simulink model "hybrid_power"  (R2024b)
settings: Solver=ode45  StartTime=0.0  StopTime=3  MaxStep=0.001  RelTol=1e-3  EnableMultiTasking=on
values from neighbouring files (symbols this model uses):
  Iph_array = Iph*Npar    (= 29.801)    [pvinput.m]
  Isat_array = Isat*Npar    (= 5.8765e-08)    [pvinput.m]
  Rp_array = Rp*Nser/Npar    (= 198.702)    [pvinput.m]
  Rs_array = Rs*Nser/Npar    (= 0.0075996)    [pvinput.m]
  Ts = Ts_Power    (= 1e-06)    [pvinput.m]
  Ts_Control = 100e-6    (= 0.0001)    [pvinput.m]
  Ts_Power = 1e-6    (= 1e-06)    [pvinput.m]
  VT_array = VT*Nser    (= 3.20466023218)    [pvinput.m]
undefined symbols (not defined in the file or in its folder): DiscIntNeverNeededParam, sigbuilder_block
libraries: spsVoltageMeasurementLib x14, spsSeriesRLCBranchLib x8, spsControlledVoltageSourceLib x8, spsGroundLib x5, spsDiodeLib x4, spsIGBTDiodeLib x4, spsParallelRLCBranchLib x3, spsCurrentMeasurementLib x2, simulink x2, spsControlledCurrentSourceLib x2, spsPWMGenerator2LevelLib x1, powerlib_extras x1
settings Model: Creator=Hasin Punno  LastModifiedBy=amank
settings SolverCC: AlgebraicLoopSolver=TrustRegion
settings DataIOCC: LimitDataPoints=on  SaveFormat=Array  SignalLoggingSaveFormat=ModelDataLogs  ReturnWorkspaceOutputs=off
settings OptimizationCC: ExpressionDepthLimit=2147483647  LifeSpan=inf
settings DebuggingCC: UnderspecifiedInitializationDetection=Classic  MergeDetectMultiDrivingBlocksExec=none  SolverPrmCheckMsg=warning  FcnCallInpInsideContextMsg=warning  UnconnectedInputMsg=warning  UnconnectedOutputMsg=warning  UnconnectedLineMsg=warning  StateNameClashWarn=warning  SFUnexpectedBacktrackingDiag=warning  SFNoUnconditionalDefaultTransitionDiag=warning  SFExecutionAtInitializationDiag=none  ArithmeticOperatorsInVariantConditions=warning
settings HardwareCC: ProdBitPerPointer=32  ProdBitPerSizeT=32  ProdBitPerPtrDiffT=32  ProdLargestAtomicFloat=None  ProdIntDivRoundTo=Undefined  ProdEndianess=Unspecified  ProdWordSize=32  ProdHWDeviceType=32-bit Generic
settings ModelReferenceCC: EnableRefExpFcnMdlSchedulingChecks=on  PropagateSignalLabelsOutOfModel=off
settings SFSimCC: SimUseLocalCustomCode=off  CustomCodeUndefinedFunction=UseInterfaceOnly
settings RTWCC: RTWUseLocalCustomCode=off  GPUComputeCapability=3.5
settings CodeAppCC: StateflowObjectComments=on
settings GRTTargetCC: TargetLangStandard=C89/C90 (ANSI)
settings ConfigComp: CovMetricSettings=dw  CovSaveCumulativeToWorkspaceVar=on  CovSaveSingleToWorkspaceVar=on  CovExternalEMLEnable=off  CovSFcnEnable=off
settings SimscapeCC: SimscapeNormalizeSystem=off

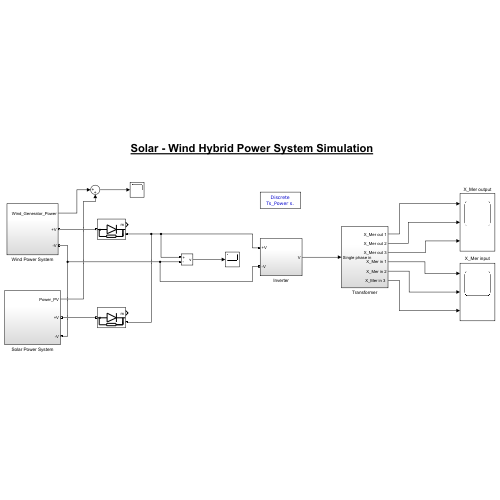
[thumbnail: Simulink's stored preview of the top-level diagram]
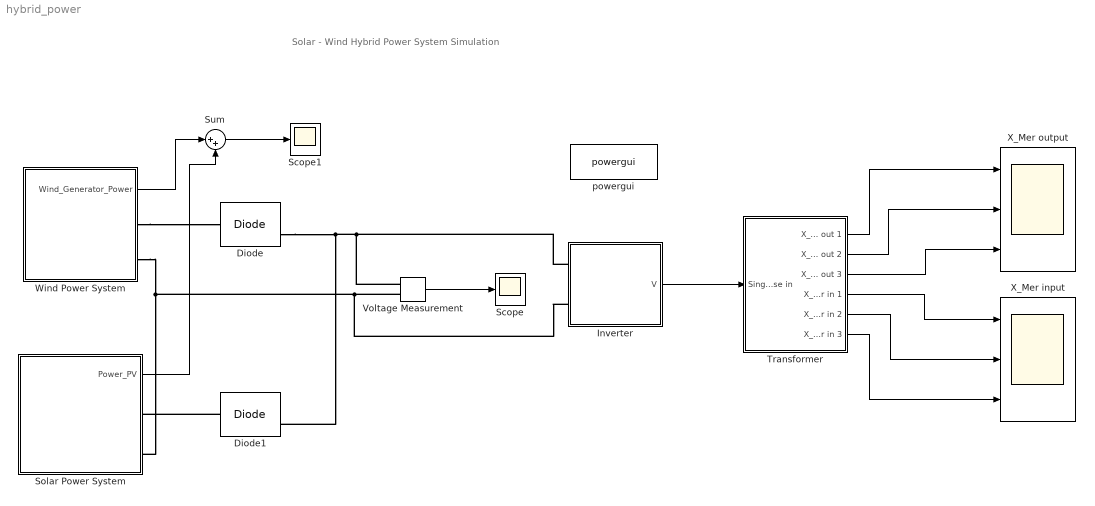
== system hybrid_power ==
  note: Solar - Wind Hybrid Power System Simulation
  Diode : spsDiodeLib/Diode  Ron=0.001  Lon=0  Vf=0.8  IC=0  UseSnubber=off  Rs=500  Cs=1e-9  Measurements=on
  Diode1 : spsDiodeLib/Diode  Ron=0.001  Lon=0  Vf=0.8  IC=0  UseSnubber=off  Rs=500  Cs=1e-9  Measurements=on
  "Inverter " : Subsystem
  Scope : Scope
  Scope1 : Scope
  "Solar Power System " : Subsystem
  Sum : Sum  Inputs=|++
  "Transformer " : Subsystem
  Voltage Measurement : spsVoltageMeasurementLib/Voltage Measurement  PhasorSimulation=off  OutputType=Complex  PSBequivalent=0
  Wind Power System : Subsystem
  X_Mer input : Scope  NumInputPorts=3
  X_Mer output : Scope  NumInputPorts=3
  powergui : spspowerguiLib/powergui  Priority=1  SimulationMode=Discrete  SampleTime=Ts_Power  frequency=60  Iterations=50  frequencyindice=0  Pbase=100e6  ErrMax=1e-4  UnitsV=kV  UnitsW=MW  buscounter=0  FunctionMessages=off  echomessages=off  EnableUseOfTLC=off  CurrentSourceSwitches=off  DisableSnubberDevices=off  DisableRonSwitches=off  DisableVfSwitches=off  DisplayEquations=off  AutomaticDiscreteSolvers=off  SolverType=Tustin  Interpol=off  ExternalGateDelay=off  methode=off  Ts=0  x0status=blocks  SPID=off  SwTol=0  HookPort=off  NonlinearTolerance=1e-4  nMaxIteration=100  ContinueOnMaxIteration=off  RestoreLinks=warning  ResistiveCurrentMeasurement=off  Frange=[0:2:500]  Ylog=off  Xlog=on  ShowGrid=off  save=off  variable=ZData  structure=0  ZoomFFT=on  StartTime=0.0  cycles=1  DisplayStyle=1  fundamental=60  FreqAxis=off  MaxFrequency=1000  frequencyindicesteady=1  RmsSteady=1  display=off
  wires:
  Voltage Measurement/1 -> Scope/1
  Wind Power System/1(Wind_Generator_Power) -> Sum/1
  "Solar Power System "/1(Power_PV) -> Sum/2
  "Inverter "/1(V) -> "Transformer "/1("Single phase in ")
  "Transformer "/1(X_Mer out 1) -> X_Mer output/1
  "Transformer "/2(X_Mer out 2) -> X_Mer output/2
  "Transformer "/3(X_Mer out 3) -> X_Mer output/3
  "Transformer "/4(X_Mer in 1) -> X_Mer input/1
  "Transformer "/5(X_Mer in 2) -> X_Mer input/2
  "Transformer "/6("X_Mer in 3 ") -> X_Mer input/3
  Sum/1 -> Scope1/1
  connections:
  Wind Power System/RConn1 -- Diode/LConn1
  Diode1/LConn1 -- "Solar Power System "/RConn1
  Diode/RConn1 -- Diode1/RConn1 -- Voltage Measurement/LConn1 -- "Inverter "/LConn1
  Wind Power System/RConn2 -- Voltage Measurement/LConn2 -- "Inverter "/LConn2 -- "Solar Power System "/RConn2

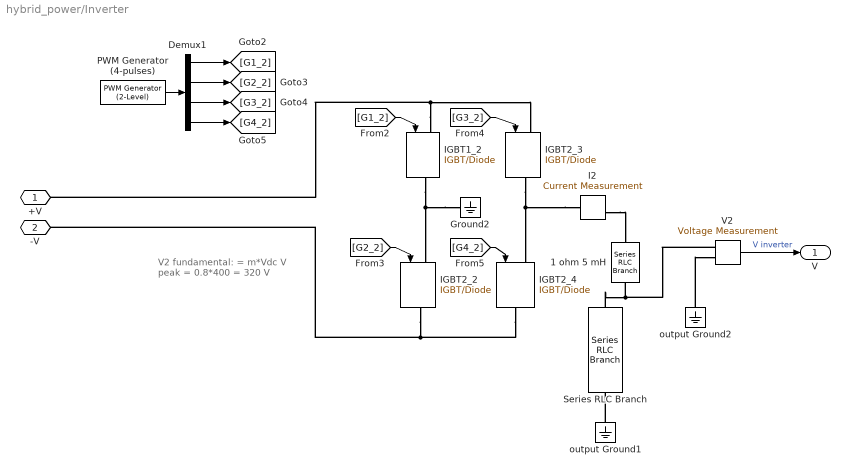
== system hybrid_power/Inverter  ==
  note: V2 fundamental:
      |     = m*Vdc V peak
      |     = 0.8*400
      |     = 320 V
  "1 ohm 5 mH " : spsSeriesRLCBranchLib/Series RLC Branch  LConnTagsString=__new0  RConnTagsString=__new0  BranchType=RL  Resistance=27  Inductance=100e-03  SetiL0=off  InitialCurrent=0  Capacitance=[]  Setx0=off  InitialVoltage=0  Measurements=None
  Demux1 : Demux
  Ground2 : spsGroundLib/Ground  LConnTagsString=a
  I2 : spsCurrentMeasurementLib/Current Measurement  Tag=PoWeRsYsTeMmEaSuReMeNt  PhasorSimulation=off  OutputType=Magnitude  PSBequivalent=0
      settings: AttributesFormatString=\n
  IGBT1_2 : spsIGBTDiodeLib/IGBT//Diode  Ron=1e-3  Rs=1e5  Cs=inf  Measurements=off
  IGBT2_2 : spsIGBTDiodeLib/IGBT//Diode  Ron=1e-3  Rs=1e5  Cs=inf  Measurements=off
  IGBT2_3 : spsIGBTDiodeLib/IGBT//Diode  Ron=1e-3  Rs=1e5  Cs=inf  Measurements=off
  IGBT2_4 : spsIGBTDiodeLib/IGBT//Diode  Ron=1e-3  Rs=1e5  Cs=inf  Measurements=off
  PWM Generator (4-pulses) : spsPWMGenerator2LevelLib/PWM Generator (2-Level)  ModulatorType=Single-phase full-bridge (4 pulses)  ModulatorMode=Unsynchronized  Fc=2000  Pc=0  nF=27  MinMax="[ -1  1 ]"  SamplingTechnique=Natural  ModulatingSignals=on  m=0.8  Freq=50  Phase=0  Ts=5.144e-6  ShowCarrierOutport=off
  Series RLC Branch : spsSeriesRLCBranchLib/Series RLC Branch  LConnTagsString=__new0  RConnTagsString=__new0  BranchType=C  Resistance=1  Inductance=1e-3  SetiL0=off  InitialCurrent=0  Capacitance=100e-6  Setx0=off  InitialVoltage=0  Measurements=None
  V2 : spsVoltageMeasurementLib/Voltage Measurement  Tag=PoWeRsYsTeMmEaSuReMeNt  PhasorSimulation=off  OutputType=Magnitude  PSBequivalent=0
  output Ground1 : spsGroundLib/Ground  LConnTagsString=a
  output Ground2 : spsGroundLib/Ground  LConnTagsString=a
  +V : PMIOPort  Side=Left
  "-V " : PMIOPort  Port=2  Side=Left
  V : Outport
  wires:
  Demux1/4 -> [G4_2]
  V2/1 -> V/1  "V inverter"
  Demux1/2 -> [G2_2]
  [G1_2] -> IGBT1_2/1
  Demux1/3 -> [G3_2]
  PWM Generator (4-pulses)/1 -> Demux1/1
  [G3_2] -> IGBT2_3/1
  Demux1/1 -> [G1_2]
  [G2_2] -> IGBT2_2/1
  [G4_2] -> IGBT2_4/1
  connections:
  I2/LConn1 -- IGBT2_3/RConn1 -- IGBT2_4/LConn1
  V2/LConn1 -- Series RLC Branch/LConn1 -- "1 ohm 5 mH "/RConn1
  Ground2/LConn1 -- IGBT1_2/RConn1 -- IGBT2_2/LConn1
  output Ground2/LConn1 -- V2/LConn2
  I2/RConn1 -- "1 ohm 5 mH "/LConn1
  IGBT1_2/LConn1 -- +V/RConn1 -- IGBT2_3/LConn1
  IGBT2_2/RConn1 -- "-V "/RConn1 -- IGBT2_4/RConn1
  output Ground1/LConn1 -- Series RLC Branch/RConn1

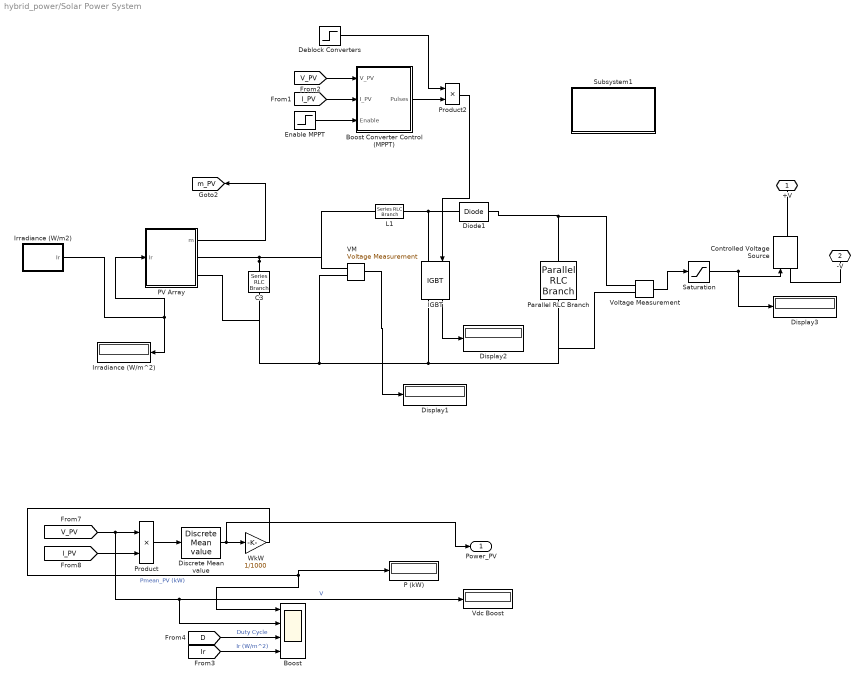
== system hybrid_power/Solar Power System  ==
  Boost : Scope  NumInputPorts=4
  Boost Converter Control (MPPT) : Subsystem
  C3 : spsSeriesRLCBranchLib/Series RLC Branch  LConnTagsString=__new0  RConnTagsString=__new0  BranchType=C  Resistance=1.0  Inductance=1.0  SetiL0=off  InitialCurrent=0  Capacitance=100e-6  Setx0=off  InitialVoltage=0  Measurements=Branch voltage
  Controlled Voltage Source : spsControlledVoltageSourceLib/Controlled Voltage Source  Initialize=on  Source_Type=AC  Amplitude=0  Phase=0  Frequency=0  Measurements=None
  Deblock Converters : Step  Time=0.05  SampleTime=0
  Diode1 : spsDiodeLib/Diode  Ron=1e-4  Lon=0  Vf=0  IC=0  UseSnubber=off  Rs=inf  Cs=inf  Measurements=off
  Discrete Mean value : powerlib_extras/Discrete Measurements/Discrete  Mean value  Freq=60  Vinit=0  Ts=Ts_Control
  Display1 : Display
  Display2 : Display
  Display3 : Display
  Enable MPPT : Step  Time=0.4  SampleTime=0
  IGBT : spsIGBTLib/IGBT  Ron=0.001  Lon=0  Vf=0  Tf=0  Tt=0  IC=0  Rs=1e5  Cs=inf  Measurements=on
  "Irradiance (W/m2) " : Subsystem  Tag=STV Subsys  LoadFcn=sigbuilder_block('load');  StartFcn=sigbuilder_block('start');  StopFcn=sigbuilder_block('stop');  ClipboardFcn=sigbuilder_block('clipboard');  mask(Sigbuilder block){tuvar=[0:10]}
      mask help: Sigbuilder GUI
      mask init:
      | if ~strcmp(get_param(bdroot(gcbh),'SimulationStatus'),'stopped') tuvar = sigbuilder_block('maskInit'); end
      settings: CopyFcn=sigbuilder_block('copy');  DeleteFcn=sigbuilder_block('delete');  ModelCloseFcn=sigbuilder_block('modelClose');  PreSaveFcn=sigbuilder_block('preSave');  PauseFcn=sigbuilder_block('pause')  ContinueFcn=sigbuilder_block('continue')  NameChangeFcn=sigbuilder_block('namechange');  OpenFcn=sigbuilder_block('open',[9 39 954 473.25 ]);  CloseFcn=sigbuilder_block('close');
      mask Display: plot(0, 0, 100, 100,[2, 2, 32, 32, 2], [68, 8, 8, 68, 68],[32, 2], [38, 38], [32, 19, 2],[53, 60, 44], [32, 17, 17, 2],[16, 16, 31, 31]);txt = getActiveGroup(gcbh);text(2, 100, txt,'verticalAlignment', 'top');
  Irradiance (W/m^2) : Display
      settings: Format=bank  Decimation=1000
  L1 : spsSeriesRLCBranchLib/Series RLC Branch  LConnTagsString=__new0  RConnTagsString=__new0  BranchType=RL  Resistance=0.005  Inductance=5e-3  SetiL0=off  InitialCurrent=0  Capacitance=1e-6  Setx0=off  InitialVoltage=0  Measurements=None
  "P (kW) " : Display
      settings: Format=bank  Decimation=2000
  PV Array : Subsystem
  Parallel RLC Branch : spsParallelRLCBranchLib/Parallel RLC Branch  LConnTagsString=a  RConnTagsString=__new0  BranchType=RC  Resistance=1e3  Inductance=1e-3  SetiL0=off  InitialCurrent=0  Capacitance=1e-6  Setx0=off  InitialVoltage=0  Measurements=None
  Product : Product  RndMeth=Zero
  Product2 : Product  RndMeth=Zero
  Saturation : Saturate  UpperLimit=48  LowerLimit=0
  Subsystem1 : Subsystem
      mask Display: disp('Measurements')
  VM : spsVoltageMeasurementLib/Voltage Measurement  PhasorSimulation=off  OutputType=Complex  PSBequivalent=0
  Vdc Boost : Display
      settings: Format=bank  Decimation=2000
  Voltage Measurement : spsVoltageMeasurementLib/Voltage Measurement  PhasorSimulation=off  OutputType=Complex  PSBequivalent=0
  WkW : Gain  Gain=1/1000
  +V : PMIOPort  Side=Right
  -V : PMIOPort  Port=2  Side=Right
  Power_PV : Outport
  tag scope: m_PV=global
  wires:
  Voltage Measurement/1 -> Saturation/1
  Saturation/1 -> Controlled Voltage Source/1, Display3/1
  IGBT/1 -> Display2/1
  PV Array/1(m) -> [m_PV]
  [D] -> Boost/3  "Duty Cycle"
  [V_PV] -> Vdc Boost/1, Boost/2, Product/1  "V"
  VM/1 -> Display1/1
  "Irradiance (W/m2) "/1(Ir) -> Irradiance (W/m^2)/1, PV Array/1(Ir)
  [Ir] -> Boost/4  "Ir (W/m^2)"
  Deblock Converters/1 -> Product2/1
  Product2/1 -> IGBT/1
  Enable MPPT/1 -> Boost Converter Control (MPPT)/3(Enable)
  Boost Converter Control (MPPT)/1(Pulses) -> Product2/2
  [I_PV] -> Boost Converter Control (MPPT)/2(I_PV)
  [V_PV] -> Boost Converter Control (MPPT)/1(V_PV)
  Discrete Mean value/1 -> Power_PV/1, WkW/1
  WkW/1 -> "P (kW) "/1, Boost/1  "Pmean_PV (kW)"
  [I_PV] -> Product/2
  Product/1 -> Discrete Mean value/1
  connections:
  Controlled Voltage Source/LConn1 -- -V/RConn1
  +V/RConn1 -- Controlled Voltage Source/RConn1
  IGBT/LConn1 -- L1/RConn1 -- Diode1/LConn1
  C3/LConn1 -- PV Array/RConn1 -- L1/LConn1 -- VM/LConn1
  VM/LConn2 -- PV Array/RConn2 -- C3/RConn1 -- IGBT/RConn1 -- Parallel RLC Branch/RConn1 -- Voltage Measurement/LConn2
  Voltage Measurement/LConn1 -- Parallel RLC Branch/LConn1 -- Diode1/RConn1

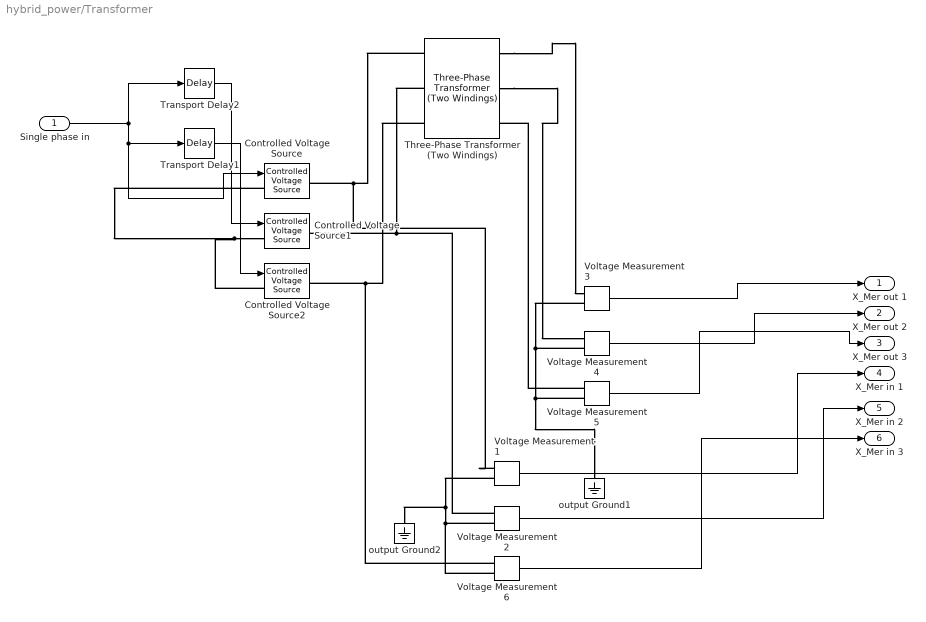
== system hybrid_power/Transformer  ==
  "Single phase in " : Inport
  Controlled Voltage Source : spsControlledVoltageSourceLib/Controlled Voltage Source  Initialize=on  Source_Type=AC  Amplitude=48  Phase=0  Frequency=50  Measurements=Voltage
  Controlled Voltage Source1 : spsControlledVoltageSourceLib/Controlled Voltage Source  Initialize=on  Source_Type=AC  Amplitude=48  Phase=120  Frequency=50  Measurements=Voltage
  Controlled Voltage Source2 : spsControlledVoltageSourceLib/Controlled Voltage Source  Initialize=on  Source_Type=AC  Amplitude=48  Phase=240  Frequency=50  Measurements=None
  Three-Phase Transformer (Two Windings) : spsThreePhaseTransformerTwoWindingsLib/Three-Phase Transformer (Two Windings)  Winding1Connection=Yg  Winding2Connection=Yg  CoreType=Three single-phase transformers  SetSaturation=off  Hysteresis=off  DataFile='hysteresis'  SetInitialFlux=off  Measurements=None  UNITS=SI  NominalPower=[9444 , 50 ]  Winding1=[48 0.018432 0.00023468]  Winding2=[460 1.62 0.020626]  Rm=4608  Lm=14.668  L0=0.5  Saturation=[0 0;0.010206 1.2475e+05;4.2526 1.5802e+05]  InitialFluxes=[83168 -83168 72773]  BreakLoop=off  DiscreteSolver=Trapezoidal iterative  DataType=on  TransfoNumber=1
  Transport Delay1 : TransportDelay  DelayTime=0.013333  BufferSize=10240
  Transport Delay2 : TransportDelay  DelayTime=6.6667e-3  BufferSize=10240
  Voltage Measurement{1..6} (6 alike) : spsVoltageMeasurementLib/Voltage Measurement  PhasorSimulation=off  OutputType=Complex  PSBequivalent=0
  output Ground1 : spsGroundLib/Ground  LConnTagsString=a
  output Ground2 : spsGroundLib/Ground  LConnTagsString=a
  X_Mer out 1 : Outport
  X_Mer out 2 : Outport  Port=2
  X_Mer out 3 : Outport  Port=3
  X_Mer in 1 : Outport  Port=4
  X_Mer in 2 : Outport  Port=5
  "X_Mer in 3 " : Outport  Port=6
  wires:
  Voltage Measurement5/1 -> X_Mer out 3/1
  Voltage Measurement4/1 -> X_Mer out 2/1
  Transport Delay1/1 -> Controlled Voltage Source2/1
  "Single phase in "/1 -> Controlled Voltage Source/1, Transport Delay1/1, Transport Delay2/1
  Transport Delay2/1 -> Controlled Voltage Source1/1
  Voltage Measurement1/1 -> X_Mer in 1/1
  Voltage Measurement6/1 -> "X_Mer in 3 "/1
  Voltage Measurement2/1 -> X_Mer in 2/1
  Voltage Measurement3/1 -> X_Mer out 1/1
  connections:
  Three-Phase Transformer (Two Windings)/RConn1 -- Voltage Measurement3/LConn1
  Controlled Voltage Source/LConn1 -- Controlled Voltage Source2/LConn1 -- Controlled Voltage Source1/LConn1
  Three-Phase Transformer (Two Windings)/LConn1 -- Voltage Measurement1/LConn1 -- Controlled Voltage Source/RConn1
  Voltage Measurement5/LConn1 -- Three-Phase Transformer (Two Windings)/RConn3
  Three-Phase Transformer (Two Windings)/RConn2 -- Voltage Measurement4/LConn1
  Three-Phase Transformer (Two Windings)/LConn2 -- Controlled Voltage Source1/RConn1 -- Voltage Measurement2/LConn1
  Voltage Measurement6/LConn2 -- Voltage Measurement1/LConn2 -- output Ground2/LConn1 -- Voltage Measurement2/LConn2
  Three-Phase Transformer (Two Windings)/LConn3 -- Voltage Measurement6/LConn1 -- Controlled Voltage Source2/RConn1
  Voltage Measurement5/LConn2 -- Voltage Measurement3/LConn2 -- Voltage Measurement4/LConn2 -- output Ground1/LConn1

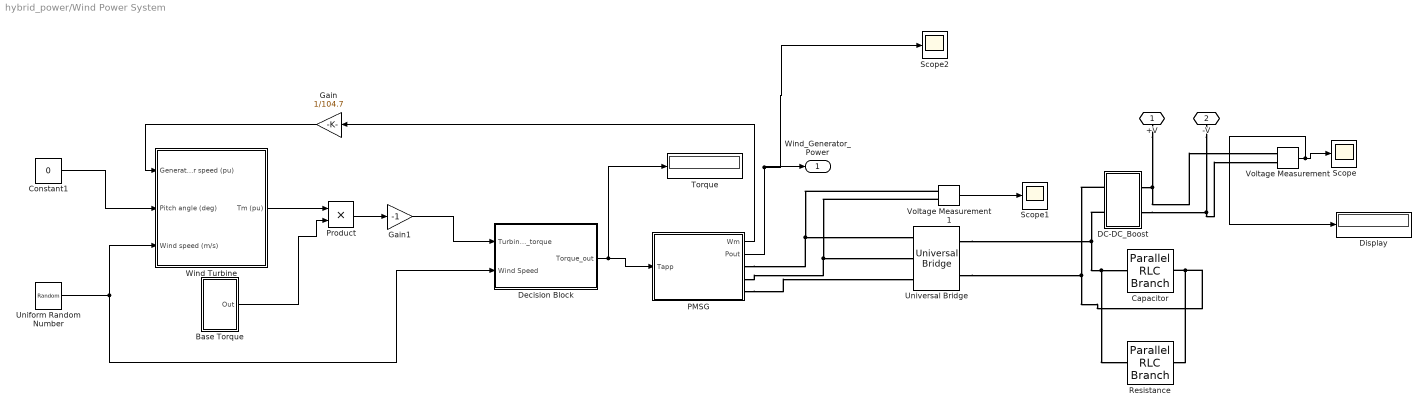
== system hybrid_power/Wind Power System ==
  Base Torque : Subsystem  mask{P=8500, w=104.7}
      mask prompts: P "Base Power"; w "Base speed (rad/s)"
  Capacitor : spsParallelRLCBranchLib/Parallel RLC Branch  LConnTagsString=a  RConnTagsString=__new0  BranchType=C  Resistance=1  Inductance=1e-3  SetiL0=off  InitialCurrent=0  Capacitance=4.8e-4  Setx0=off  InitialVoltage=0  Measurements=None
  Constant1 : Constant  Value=0
  DC-DC_Boost : Subsystem
  Decision Block : Subsystem
  Display : Display
  Gain : Gain  Gain=1/104.7
  Gain1 : Gain  Gain=-1
  PMSG : Subsystem  mask{f=50, p=6, Xs=1, Nc=30, loss=1000, phi=0.0207862}
      mask prompts: f "Frequency(Hz)"; p "Pole"; Xs "Synchronous Reactance(Ohm)"; Nc "Number of turns"; loss "Mechanical Loss(Watt)"; phi "field(Wb-m^2)"
  Product : Product
  Resistance : spsParallelRLCBranchLib/Parallel RLC Branch  LConnTagsString=a  RConnTagsString=__new0  BranchType=R  Resistance=1000  Inductance=1e-3  SetiL0=off  InitialCurrent=0  Capacitance=1  Setx0=off  InitialVoltage=0  Measurements=None
  Scope : Scope
  Scope1 : Scope
  Scope2 : Scope
  Torque : Display
  Uniform Random Number : UniformRandomNumber  Minimum=12  Maximum=13  SampleTime=0.01
  Universal Bridge : spsUniversalBridgeLib/Universal Bridge  Arms=3  SnubberResistance=1e5  SnubberCapacitance=inf  Device=Diodes  Ron=1e-3  Lon=0  ForwardVoltages="[  0  0  ]"  ForwardVoltage=0  GTOparameters=[ 10e-6 , 20e-6 ]  IGBTparameters=[ 1e-6 , 2e-6 ]  Measurements=None  Measurements_2=None  converterType=Rectifier
  Voltage Measurement : spsVoltageMeasurementLib/Voltage Measurement  PhasorSimulation=off  OutputType=Complex  PSBequivalent=0
  Voltage Measurement1 : spsVoltageMeasurementLib/Voltage Measurement  PhasorSimulation=off  OutputType=Complex  PSBequivalent=0
  Wind Turbine : Subsystem  AncestorBlock=re_lib/Wind Generation/Wind Turbine  DialogController=POWERSYS.PowerSysDialog  mask(Wind Turbine){Pnom=8500, Pelec_base=8500/0.9, wind_base=12, P_wind_base=0.8, speed_nom=1, pitch_angle=0, c1_c6=[0.51763          116          0.4            5           21     0.006795], cp_nom=0.48, lambda_nom=8.1}
      mask prompts: Pnom "Nominal mechanical output power (W):"; Pelec_base "Base power of the electrical generator (VA):"; wind_base "Base wind speed (m/s):"; P_wind_base "Maximum power at base wind speed (pu of nominal mechanical power):"; speed_nom "Base rotational speed (p.u. of base generator speed):"; pitch_angle "Pitch angle beta to display wind-turbine power characteristics (beta >=0)  (deg):"
      mask help:
      | This block implements a variable pitch wind turbine model. The performance coefficient Cp of the turbine is the mechanical output power of the turbine divided by wind power and a function of wind speed, rotational speed, and pitch angle (beta). Cp reaches its maximum value at zero beta. Select the wind-turbine power characteristics display to plot the turbine characteristics at the specified pitch angle.
      |
      | The first input is the generator speed in per unit of the generator base speed. For a synchronous or asynchronous generator, the base speed is the synchronous speed. For a permanent-magnet generator, the base speed is defined as the speed producing nominal voltage at  no load. The second input is the blade pitch angle (beta) in degrees. The third input is the wind speed in m/s.
      |
      | The output is the torque applied to the generator shaft in per unit of the generator ratings.
      |
      | The turbine inertia must be added to the generator inertia.
      mask init:
      | c1=c1_c6(1);c2=c1_c6(2);c3=c1_c6(3);c4=c1_c6(4);c5=c1_c6(5);c6=c1_c6(6);
      | if ~(wind_base>0)
      |     error(message('physmod:powersys:common:GreaterThan',getfullname(gcbh),'Base wind speed (m/s)',0));
      | end
      | 
      | power_initmask();
      mask Help: helpview(psbhelp);
      mask DialogControl DisplayTurbChar Prompt: Display wind turbine power characteristics
      mask DialogControl DisplayTurbChar Callback: WindTurbinePlot(gcb)
      mask Display: disp('');
  +V : PMIOPort  Side=Right
  -V : PMIOPort  Port=2  Side=Right
  Wind_Generator_Power : Outport
  wires:
  Gain/1 -> Wind Turbine/1(Generator speed (pu))
  Voltage Measurement/1 -> Display/1, Scope/1
  Base Torque/1(Out) -> Product/2
  Product/1 -> Gain1/1
  PMSG/1(Wm) -> Gain/1
  Wind Turbine/1(Tm (pu)) -> Product/1
  Decision Block/1(Torque_out) -> Torque/1, PMSG/1(Tapp)
  Gain1/1 -> Decision Block/1(Turbine_torque)
  Voltage Measurement1/1 -> Scope1/1
  Constant1/1 -> Wind Turbine/2(Pitch angle (deg))
  PMSG/2(Pout) -> Scope2/1, Wind_Generator_Power/1
  Uniform Random Number/1 -> Decision Block/2(Wind Speed), Wind Turbine/3(Wind speed (m/s))
  connections:
  DC-DC_Boost/RConn1 -- Voltage Measurement/LConn1 -- +V/RConn1
  DC-DC_Boost/RConn2 -- Voltage Measurement/LConn2 -- -V/RConn1
  Universal Bridge/RConn1 -- Capacitor/LConn1 -- Resistance/LConn1 -- DC-DC_Boost/LConn2
  Universal Bridge/RConn2 -- Resistance/RConn1 -- Capacitor/RConn1 -- DC-DC_Boost/LConn1
  PMSG/RConn1 -- Voltage Measurement1/LConn1 -- Universal Bridge/LConn1
  PMSG/RConn2 -- Voltage Measurement1/LConn2 -- Universal Bridge/LConn2
  PMSG/RConn3 -- Universal Bridge/LConn3

== system hybrid_power/Solar Power System /Boost Converter Control (MPPT) ==
  V_PV : Inport
  I_PV : Inport  Port=2
  Enable : Inport  Port=3
  Add : Sum  Inputs=+-
  Initial Duty Cycle : Constant  Value=0.5
  MPPT : Subsystem
  Pulse Generator : Subsystem  mask{Freq=5000}
      mask prompts: Freq "Frequency (Hz)"
  Saturation : Saturate  UpperLimit=1  LowerLimit=0
  Pulses : Outport
  tag scope: D=global
  wires:
  Initial Duty Cycle/1 -> Add/1
  MPPT/1(Delta_D) -> Add/2
  Add/1 -> Saturation/1  "D"
  Saturation/1 -> Pulse Generator/1(D), [D]
  Enable/1 -> MPPT/3(on/off)
  Pulse Generator/1(Pulses) -> Pulses/1
  I_PV/1 -> MPPT/2(I_PV)
  V_PV/1 -> MPPT/1(V_PV)

== system hybrid_power/Solar Power System /Irradiance (W//m2)  ==
  Demux : Demux  Tag=STV Demux  Outputs=1
      settings: DisplayOption=none
  FromWs : FromWorkspace  Tag=STV FromWs  VariableName=tuvar
      SigBuilderData=|
      | common.afterFinalStr = 'Extrapolate'
      | common.sampleTime = '0'
      | dataSet(1).timeRange = [0 1]
      | dataSet(1).name = 'Constant Irradiance'
      | dataSet(2).timeRange = [0 1]
      | dataSet(2).name = 'Step Irradiance'
      | dataSet(3).timeRange = [0 3]
      | dataSet(3).name = 'Ramp-up/down Irradiance'
      | sbobj.Groups(1).Name = 'Constant Irradiance'
      | sbobj.Groups(1).Signals.Name = 'Ir'
      | sbobj.Groups(1).Signals.XData = [0 1]
      | sbobj.Groups(1).Signals.YData = [1000 1000]
      | sbobj.Groups(1).TimeRange = [0 1]
      | sbobj.Groups(2).Name = 'Step Irradiance'
      | sbobj.Groups(2).Signals.Name = 'Ir'
      | sbobj.Groups(2).Signals.XData = [0 0.501 0.51 0.69 0.7 1]
      | sbobj.Groups(2).Signals.YData = [1000 1000 250 250 1000 1000]
      | sbobj.Groups(2).TimeRange = [0 1]
      | sbobj.Groups(3).Name = 'Ramp-up/down Irradiance'
      | sbobj.Groups(3).Signals.Name = 'Ir'
      | sbobj.Groups(3).Signals.XData = [0 0.7 1.2 1.2 1.5 2 2.3 2.35 2.65 2.7 3]
      | sbobj.Groups(3).Signals.YData = [1000 1000 590 595 595 1000 1000 250 250 1000 1000]
      | sbobj.Groups(3).TimeRange = [0 3]
  Ir : Outport  Tag=STV Outport
  wires:
  Demux/1 -> Ir/1
  FromWs/1 -> Demux/1

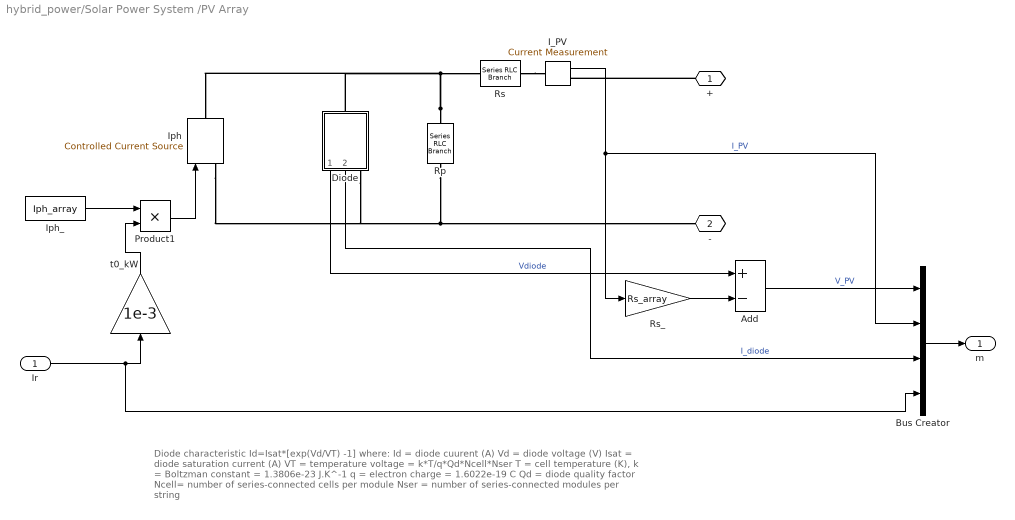
== system hybrid_power/Solar Power System /PV Array ==
  note: Diode characteristic
      | Id=Isat*[exp(Vd/VT) -1]
      |
      | where:
      | Id = diode cuurent (A)
      | Vd = diode voltage (V)
      | Isat = diode saturation current (A)
      | VT = temperature voltage = k*T/q*Qd*Ncell*Nser
      |
      | T = cell temperature (K),
      | k = Boltzman constant = 1.3806e-23 J.K^-1
      | q = electron charge = 1.6022e-19 C
      | Qd = diode quality factor
      | Ncell= number of series-connected cells per module
      | Nser = number of series-connected modules per string
  Ir : Inport
  Add : Sum  Inputs=+-
  Bus Creator : BusCreator  Inputs=4
  Diode : Subsystem
      mask Display:
      | plot(-75,-50,100,150, [-15 -15 43 -15 -15 -75],[50 8 50 92 50 50], ...
      |     [43 43],[8 94],[100 43], [50 50])
  I_PV : spsCurrentMeasurementLib/Current Measurement  PhasorSimulation=off  OutputType=Complex  PSBequivalent=0
  Iph : spsControlledCurrentSourceLib/Controlled Current Source  Initialize=on  Source_Type=AC  Amplitude=0  Phase=0  Frequency=0  Measurements=None
  Iph_ : Constant  Value=Iph_array
  Product1 : Product  Inputs=**  RndMeth=Zero
  Rp : spsSeriesRLCBranchLib/Series RLC Branch  LConnTagsString=__new0  RConnTagsString=__new0  BranchType=R  Resistance=Rp_array  Inductance=1e-3  SetiL0=off  InitialCurrent=0  Capacitance=1e-6  Setx0=off  InitialVoltage=0  Measurements=Branch current
  Rs : spsSeriesRLCBranchLib/Series RLC Branch  LConnTagsString=__new0  RConnTagsString=__new0  BranchType=R  Resistance=Rs_array  Inductance=1e-3  SetiL0=off  InitialCurrent=0  Capacitance=1e-6  Setx0=off  InitialVoltage=0  Measurements=None
  Rs_ : Gain  Gain=Rs_array
  t0_kW : Gain  Gain=1e-3
  + : PMIOPort  Side=Right
  - : PMIOPort  Port=2  Side=Right
  m : Outport
  wires:
  I_PV/1 -> Bus Creator/2, Rs_/1  "I_PV"
  Bus Creator/1 -> m/1
  Rs_/1 -> Add/2
  Diode/1(Vdiode) -> Add/1  "Vdiode"
  Diode/2(Idiode) -> Bus Creator/3  "I_diode"
  Add/1 -> Bus Creator/1  "V_PV"
  t0_kW/1 -> Product1/2
  Product1/1 -> Iph/1
  Iph_/1 -> Product1/1
  Ir/1 -> Bus Creator/4, t0_kW/1
  connections:
  +/RConn1 -- I_PV/RConn1
  Rs/LConn1 -- I_PV/LConn1
  Rp/LConn1 -- Rs/RConn1 -- Iph/RConn1 -- Diode/LConn1
  Rp/RConn1 -- Diode/RConn1 -- Iph/LConn1 -- -/RConn1

== system hybrid_power/Solar Power System /Subsystem1 ==
  Bus Selector : BusSelector  OutputSignals=V_PV,I_PV,I_diode,signal4
  PV : Scope  NumInputPorts=3
  tag scope: I_PV=global, Idiode_PV=global, Ir=global, V_PV=global
  wires:
  [V_PV] -> PV/1  "V_PV"
  [I_PV] -> PV/2  "I_PV"
  [Idiode_PV] -> PV/3  "Idiode_PV"
  [m_PV] -> Bus Selector/1
  Bus Selector/1 -> [V_PV]  "<V_PV>"
  Bus Selector/2 -> [I_PV]  "<I_PV>"
  Bus Selector/3 -> [Idiode_PV]  "<I_diode>"
  Bus Selector/4 -> [Ir]  "<signal4>"

== system hybrid_power/Wind Power System/Base Torque ==
  Base Power : Constant  Value=P
  Base speed(rad/s) : Constant  Value=w
  Divide : Product  Inputs=*/
  Out : Outport
  wires:
  Divide/1 -> Out/1
  Base speed(rad/s)/1 -> Divide/2
  Base Power/1 -> Divide/1

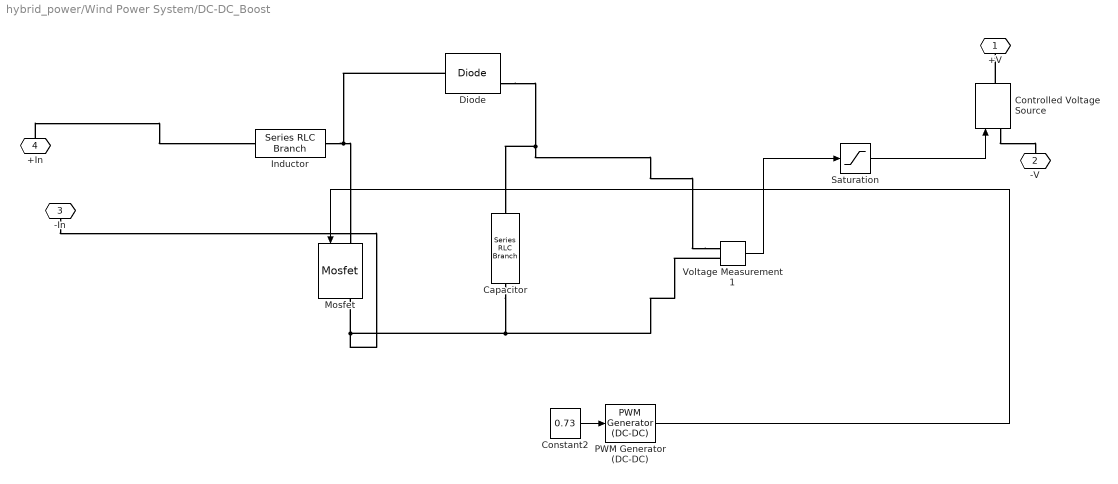
== system hybrid_power/Wind Power System/DC-DC_Boost ==
  Capacitor : spsSeriesRLCBranchLib/Series RLC Branch  LConnTagsString=__new0  RConnTagsString=__new0  BranchType=C  Resistance=1  Inductance=1e-3  SetiL0=off  InitialCurrent=0  Capacitance=33e-6  Setx0=off  InitialVoltage=0  Measurements=None
  Constant2 : Constant  Value=0.73
  Controlled Voltage Source : spsControlledVoltageSourceLib/Controlled Voltage Source  Initialize=on  Source_Type=AC  Amplitude=0  Phase=0  Frequency=0  Measurements=None
  Diode : spsDiodeLib/Diode  Ron=0.001  Lon=0  Vf=0.8  IC=0  UseSnubber=off  Rs=500  Cs=250e-9  Measurements=on
  Inductor : spsSeriesRLCBranchLib/Series RLC Branch  LConnTagsString=__new0  RConnTagsString=__new0  BranchType=L  Resistance=1  Inductance=1e-3  SetiL0=off  InitialCurrent=0  Capacitance=1e-6  Setx0=off  InitialVoltage=0  Measurements=None
  Mosfet : spsMosfetLib/Mosfet  Ron=0.001  Lon=0  Rd=0.001  Vfd=0  IC=0  Rs=1e5  Cs=inf  Measurements=on
  PWM Generator (DC-DC) : spsPWMGeneratorDCDCLib/PWM Generator (DC-DC)  Fsw=25000  Ts=0
  Saturation : Saturate  UpperLimit=48  LowerLimit=0
  Voltage Measurement1 : spsVoltageMeasurementLib/Voltage Measurement  PhasorSimulation=off  OutputType=Complex  PSBequivalent=0
  +V : PMIOPort  Side=Right
  -V : PMIOPort  Port=2  Side=Right
  -In : PMIOPort  Port=3  Side=Left
  +In : PMIOPort  Port=4  Side=Left
  wires:
  Saturation/1 -> Controlled Voltage Source/1
  Constant2/1 -> PWM Generator (DC-DC)/1
  Voltage Measurement1/1 -> Saturation/1
  PWM Generator (DC-DC)/1 -> Mosfet/1
  connections:
  Inductor/RConn1 -- Mosfet/LConn1 -- Diode/LConn1
  +In/RConn1 -- Inductor/LConn1
  Mosfet/RConn1 -- Voltage Measurement1/LConn2 -- Capacitor/RConn1 -- -In/RConn1
  Voltage Measurement1/LConn1 -- Capacitor/LConn1 -- Diode/RConn1
  Controlled Voltage Source/LConn1 -- -V/RConn1
  Controlled Voltage Source/RConn1 -- +V/RConn1

== system hybrid_power/Wind Power System/Decision Block ==
  Turbine_torque : Inport
  Wind Speed : Inport  Port=2
  Switch : Switch  Criteria=u2 > Threshold  SaturateOnIntegerOverflow=off  InputSameDT=off
  Switch1 : Switch  Criteria=u2 > Threshold  Threshold=30  SaturateOnIntegerOverflow=off  InputSameDT=off
  zero : Constant  Value=0
  Torque_out : Outport
  wires:
  Switch1/1 -> Torque_out/1
  Switch/1 -> Switch1/3
  Turbine_torque/1 -> Switch/1, Switch/2
  zero/1 -> Switch1/1, Switch/3
  Wind Speed/1 -> Switch1/2

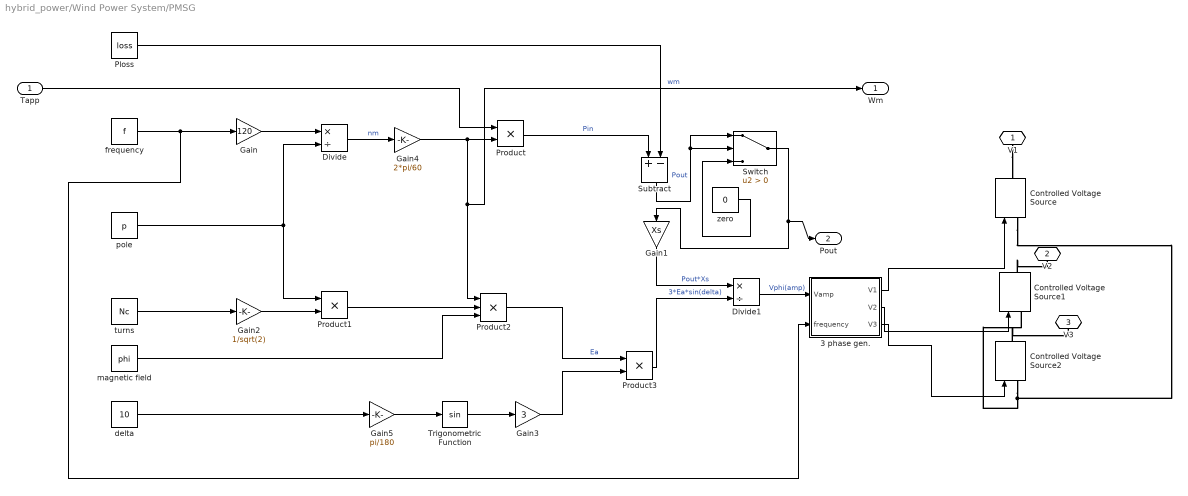
== system hybrid_power/Wind Power System/PMSG ==
  Tapp : Inport
  3 phase gen. : Subsystem
  Controlled Voltage Source : spsControlledVoltageSourceLib/Controlled Voltage Source  Initialize=on  Source_Type=AC  Amplitude=0  Phase=0  Frequency=0  Measurements=None
  Controlled Voltage Source1 : spsControlledVoltageSourceLib/Controlled Voltage Source  Initialize=on  Source_Type=AC  Amplitude=0  Phase=0  Frequency=0  Measurements=None
  Controlled Voltage Source2 : spsControlledVoltageSourceLib/Controlled Voltage Source  Initialize=on  Source_Type=AC  Amplitude=0  Phase=0  Frequency=0  Measurements=None
  Divide : Product  Inputs=*/
  Divide1 : Product  Inputs=*/
  Gain : Gain  Gain=120
  Gain1 : Gain  Gain=Xs
  Gain2 : Gain  Gain=1/sqrt(2)
  Gain3 : Gain  Gain=3
  Gain4 : Gain  Gain=2*pi/60
  Gain5 : Gain  Gain=pi/180
  Ploss : Constant  Value=loss
  Product : Product  RndMeth=Zero
  Product1 : Product  RndMeth=Zero
  Product2 : Product  Inputs=3  RndMeth=Zero
  Product3 : Product  RndMeth=Zero
  Subtract : Sum  Inputs=+-
  Switch : Switch  Criteria=u2 > Threshold  SaturateOnIntegerOverflow=off  InputSameDT=off
  Trigonometric Function : Trigonometry
  delta : Constant  Value=10
  frequency : Constant  Value=f
  magnetic field : Constant  Value=phi
  pole : Constant  Value=p
  turns : Constant  Value=Nc
  zero : Constant  Value=0
  V1 : PMIOPort  Side=Right
  V2 : PMIOPort  Port=2  Side=Right
  V3 : PMIOPort  Port=3  Side=Right
  Wm : Outport
  Pout : Outport  Port=2
  wires:
  Gain/1 -> Divide/1
  turns/1 -> Gain2/1
  Gain2/1 -> Product1/2
  Product1/1 -> Product2/2
  Trigonometric Function/1 -> Gain3/1
  Gain3/1 -> Product3/2
  Gain1/1 -> Divide1/1  "Pout*Xs"
  Product3/1 -> Divide1/2  "3*Ea*sin(delta)"
  delta/1 -> Gain5/1
  Gain5/1 -> Trigonometric Function/1
  Divide/1 -> Gain4/1  "nm"
  frequency/1 -> Gain/1, 3 phase gen./2(frequency)
  Gain4/1 -> Product/2, Product2/1, Wm/1  "wm"
  Tapp/1 -> Product/1
  pole/1 -> Divide/2, Product1/1
  Product/1 -> Subtract/1  "Pin"
  Ploss/1 -> Subtract/2
  Subtract/1 -> Switch/1, Switch/2  "Pout"
  magnetic field/1 -> Product2/3
  Product2/1 -> Product3/1  "Ea"
  Divide1/1 -> 3 phase gen./1(Vamp)  "Vphi(amp)"
  3 phase gen./1(V1) -> Controlled Voltage Source/1
  3 phase gen./2(V2) -> Controlled Voltage Source1/1
  3 phase gen./3(V3) -> Controlled Voltage Source2/1
  zero/1 -> Switch/3
  Switch/1 -> Pout/1, Gain1/1
  connections:
  Controlled Voltage Source2/LConn1 -- Controlled Voltage Source/LConn1 -- Controlled Voltage Source1/LConn1
  V1/RConn1 -- Controlled Voltage Source/RConn1
  Controlled Voltage Source1/RConn1 -- V2/RConn1
  Controlled Voltage Source2/RConn1 -- V3/RConn1

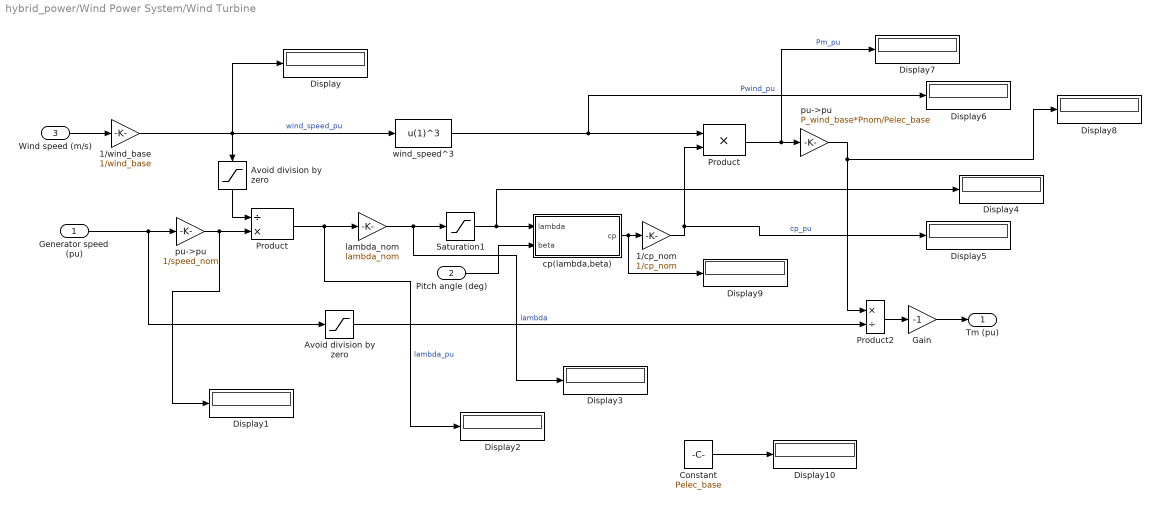
== system hybrid_power/Wind Power System/Wind Turbine ==
  Generator speed (pu) : Inport
  Pitch angle (deg) : Inport  Port=2
  Wind speed (m/s) : Inport  Port=3
  1/cp_nom : Gain  Gain=1/cp_nom  SaturateOnIntegerOverflow=on  OutDataTypeStr=Inherit: Same as input  ParamDataTypeStr=Inherit: Same as input
  1/wind_base : Gain  Gain=1/wind_base  SaturateOnIntegerOverflow=on  OutDataTypeStr=Inherit: Same as input  ParamDataTypeStr=Inherit: Same as input
  Avoid division by zero : Saturate  UpperLimit=1e6  LowerLimit=1e-6
  "Avoid division by zero " : Saturate  UpperLimit=1e6  LowerLimit=1e-6
  Constant : Constant  Value=Pelec_base
  Display{,1..10} (11 alike) : Display
  Gain : Gain  Gain=-1  SaturateOnIntegerOverflow=on  OutDataTypeStr=Inherit: Same as input  ParamDataTypeStr=Inherit: Same as input
  Product : Product  Inputs=/*  SaturateOnIntegerOverflow=on  OutDataTypeStr=Inherit: Same as first input
  "Product " : Product  SaturateOnIntegerOverflow=on  OutDataTypeStr=Inherit: Same as first input
  Product2 : Product  Inputs=*/  InputSameDT=on  SaturateOnIntegerOverflow=on  OutDataTypeStr=Inherit: Same as first input
  Saturation1 : Saturate  UpperLimit=inf  LowerLimit=1e-6
  cp(lambda,beta) : Subsystem
  lambda_nom : Gain  Gain=lambda_nom  SaturateOnIntegerOverflow=on  OutDataTypeStr=Inherit: Same as input  ParamDataTypeStr=Inherit: Same as input
  pu->pu : Gain  Gain=P_wind_base*Pnom/Pelec_base  SaturateOnIntegerOverflow=on  OutDataTypeStr=Inherit: Same as input  ParamDataTypeStr=Inherit: Same as input
  "pu->pu " : Gain  Gain=1/speed_nom  SaturateOnIntegerOverflow=on  OutDataTypeStr=Inherit: Same as input  ParamDataTypeStr=Inherit: Same as input
  wind_speed^3 : Fcn  Expr=u(1)^3
  Tm (pu) : Outport
  wires:
  Pitch angle (deg)/1 -> cp(lambda,beta)/2(beta)
  pu->pu/1 -> Display8/1, Product2/1
  cp(lambda,beta)/1(cp) -> Display9/1, 1/cp_nom/1
  wind_speed^3/1 -> Display6/1, "Product "/1  "Pwind_pu"
  Product2/1 -> Gain/1
  Avoid division by zero/1 -> Product2/2
  Wind speed (m/s)/1 -> 1/wind_base/1
  Gain/1 -> Tm (pu)/1
  Generator speed (pu)/1 -> Avoid division by zero/1, "pu->pu "/1
  "Product "/1 -> Display7/1, pu->pu/1  "Pm_pu"
  lambda_nom/1 -> Display3/1, Saturation1/1  "lambda"
  1/cp_nom/1 -> Display5/1, "Product "/2  "cp_pu"
  Saturation1/1 -> Display4/1, cp(lambda,beta)/1(lambda)
  Product/1 -> Display2/1, lambda_nom/1  "lambda_pu"
  1/wind_base/1 -> Display/1, wind_speed^3/1, "Avoid division by zero "/1  "wind_speed_pu"
  "Avoid division by zero "/1 -> Product/1
  "pu->pu "/1 -> Display1/1, Product/2
  Constant/1 -> Display10/1

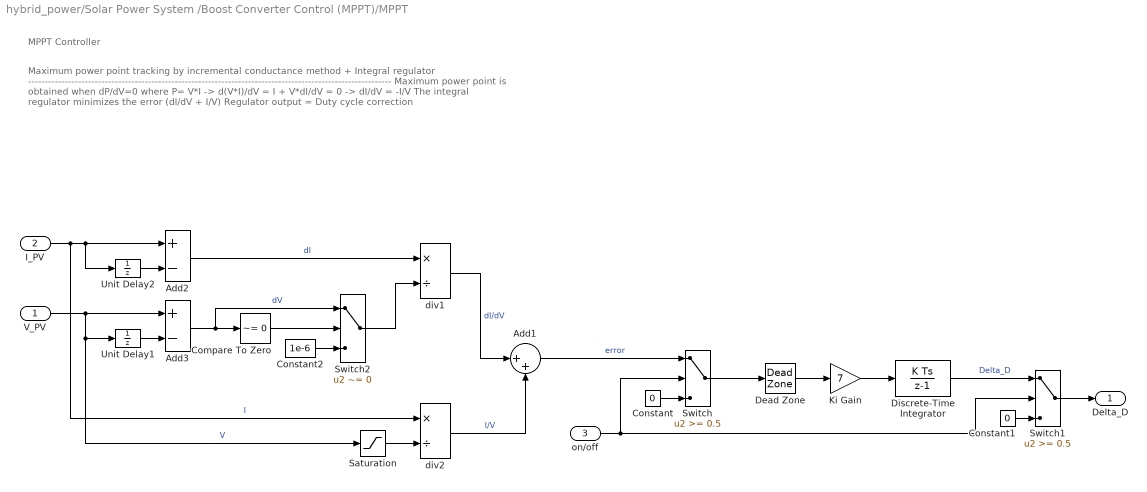
== system hybrid_power/Solar Power System /Boost Converter Control (MPPT)/MPPT ==
  note: Maximum power point tracking by incremental conductance method + Integral regulator
      | -------------------------------------------------------------------------------------------------------------
      | Maximum power point is obtained when dP/dV=0  where P= V*I
      | -> d(V*I)/dV = I + V*dI/dV = 0
      | -> dI/dV = -I/V
      | The integral regulator minimizes the error (dI/dV + I/V)
      | Regulator output = Duty cycle correction
  note: MPPT Controller
  V_PV : Inport
  I_PV : Inport  Port=2
  on/off : Inport  Port=3
  Add1 : Sum  Inputs=|++
  Add2 : Sum  Inputs=+-
  Add3 : Sum  Inputs=+-
  Compare To Zero : simulink/Logic and Bit Operations/Compare To Zero  relop=~=  OutDataTypeStr=uint8
  Constant : Constant  Value=0
  Constant1 : Constant  Value=0
  Constant2 : Constant  Value=1e-6
  Dead Zone : DeadZone  LowerValue=-0.02  UpperValue=+0.02
  Discrete-Time Integrator : DiscreteIntegrator  gainval=1  SampleTime=Ts_Control  LimitOutput=on  UpperSaturationLimit=1  LowerSaturationLimit=-1  ICPrevOutput=DiscIntNeverNeededParam  ICPrevScaledInput=DiscIntNeverNeededParam
  Ki Gain : Gain  Gain=7
  Saturation : Saturate  UpperLimit=inf  LowerLimit=eps
  Switch : Switch  Threshold=0.5  SaturateOnIntegerOverflow=off  InputSameDT=off
  Switch1 : Switch  Threshold=0.5  SaturateOnIntegerOverflow=off  InputSameDT=off
  Switch2 : Switch  Criteria=u2 ~= 0  SaturateOnIntegerOverflow=off  InputSameDT=off
  Unit Delay1 : UnitDelay  SampleTime=Ts_Control  HasFrameUpgradeWarning=on
  Unit Delay2 : UnitDelay  SampleTime=Ts_Control  HasFrameUpgradeWarning=on
  div1 : Product  Inputs=*/  RndMeth=Zero
  div2 : Product  Inputs=*/  RndMeth=Zero
  Delta_D : Outport
  wires:
  V_PV/1 -> Add3/1, Saturation/1, Unit Delay1/1  "V"
  div1/1 -> Add1/1  "dI/dV"
  Constant/1 -> Switch/3
  Switch/1 -> Dead Zone/1
  Unit Delay1/1 -> Add3/2
  Compare To Zero/1 -> Switch2/2
  Switch2/1 -> div1/2
  Constant2/1 -> Switch2/3
  I_PV/1 -> Unit Delay2/1, Add2/1, div2/1  "I"
  Unit Delay2/1 -> Add2/2
  Add3/1 -> Compare To Zero/1, Switch2/1  "dV"
  Add2/1 -> div1/1  "dI"
  Saturation/1 -> div2/2
  div2/1 -> Add1/2  "I/V"
  Add1/1 -> Switch/1  "error"
  Dead Zone/1 -> Ki Gain/1
  Constant1/1 -> Switch1/3
  Discrete-Time Integrator/1 -> Switch1/1  "Delta_D"
  Switch1/1 -> Delta_D/1
  on/off/1 -> Switch/2, Switch1/2
  Ki Gain/1 -> Discrete-Time Integrator/1

== system hybrid_power/Solar Power System /Boost Converter Control (MPPT)/Pulse Generator ==
  D : Inport
  Relational Operator : RelationalOperator  Operator=<=  OutDataTypeStr=boolean  InputSameDT=off
  Repeating Sequence : simulink/Sources/Repeating Sequence  rep_seq_t="[0  1/Freq]"  rep_seq_y=[0 1]
  Pulses : Outport
  wires:
  D/1 -> Relational Operator/2
  Relational Operator/1 -> Pulses/1
  Repeating Sequence/1 -> Relational Operator/1

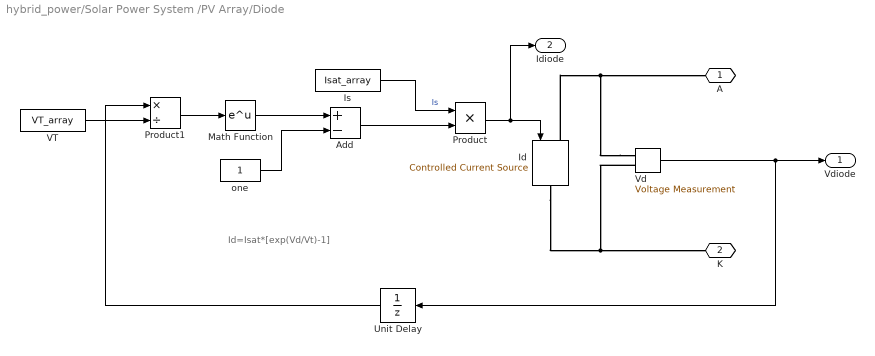
== system hybrid_power/Solar Power System /PV Array/Diode ==
  note: Id=Isat*[exp(Vd/Vt)-1]
  Add : Sum  Inputs=+-
  Id : spsControlledCurrentSourceLib/Controlled Current Source  Initialize=on  Source_Type=AC  Amplitude=0  Phase=0  Frequency=0  Measurements=None
  Is : Constant  Value=Isat_array
  Math Function : Math  SignedPower=on
  Product : Product  RndMeth=Zero
  Product1 : Product  Inputs=*/  RndMeth=Zero
  Unit Delay : UnitDelay  SampleTime=Ts  HasFrameUpgradeWarning=on
  VT : Constant  Value=VT_array
  Vd : spsVoltageMeasurementLib/Voltage Measurement  PhasorSimulation=off  OutputType=Complex  PSBequivalent=0
  one : Constant
  A : PMIOPort  Side=Left
  K : PMIOPort  Port=2  Side=Right
  Vdiode : Outport
  Idiode : Outport  Port=2
  wires:
  Product/1 -> Idiode/1, Id/1
  Vd/1 -> Vdiode/1, Unit Delay/1
  Is/1 -> Product/1  "Is"
  Product1/1 -> Math Function/1
  one/1 -> Add/2
  Add/1 -> Product/2
  VT/1 -> Product1/2
  Unit Delay/1 -> Product1/1
  Math Function/1 -> Add/1
  connections:
  Id/RConn1 -- K/RConn1 -- Vd/LConn2
  Vd/LConn1 -- A/RConn1 -- Id/LConn1

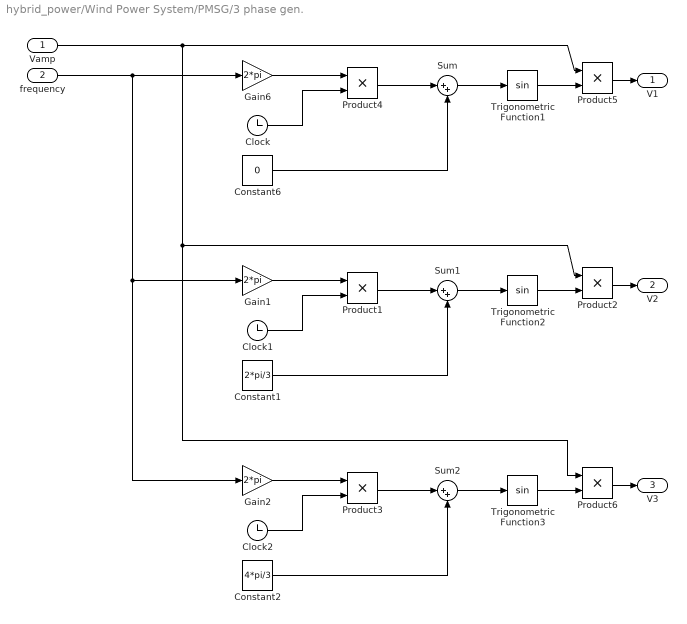
== system hybrid_power/Wind Power System/PMSG/3 phase gen. ==
  Vamp : Inport
  frequency : Inport  Port=2
  Clock : Clock
  Clock1 : Clock
  Clock2 : Clock
  Constant1 : Constant  Value=2*pi/3
  Constant2 : Constant  Value=4*pi/3
  Constant6 : Constant  Value=0
  Gain1 : Gain  Gain=2*pi
  Gain2 : Gain  Gain=2*pi
  Gain6 : Gain  Gain=2*pi
  Product{1..6} (6 alike) : Product  RndMeth=Zero
  Sum : Sum  Inputs=|++
  Sum1 : Sum  Inputs=|++
  Sum2 : Sum  Inputs=|++
  Trigonometric Function1 : Trigonometry
  Trigonometric Function2 : Trigonometry
  Trigonometric Function3 : Trigonometry
  V1 : Outport
  V2 : Outport  Port=2
  V3 : Outport  Port=3
  wires:
  Trigonometric Function1/1 -> Product5/2
  Product4/1 -> Sum/1
  Sum/1 -> Trigonometric Function1/1
  Clock/1 -> Product4/2
  Constant6/1 -> Sum/2
  Gain6/1 -> Product4/1
  frequency/1 -> Gain6/1, Gain1/1, Gain2/1
  Product5/1 -> V1/1
  Trigonometric Function2/1 -> Product2/2
  Product1/1 -> Sum1/1
  Sum1/1 -> Trigonometric Function2/1
  Clock1/1 -> Product1/2
  Constant1/1 -> Sum1/2
  Gain1/1 -> Product1/1
  Product2/1 -> V2/1
  Trigonometric Function3/1 -> Product6/2
  Product3/1 -> Sum2/1
  Sum2/1 -> Trigonometric Function3/1
  Clock2/1 -> Product3/2
  Constant2/1 -> Sum2/2
  Gain2/1 -> Product3/1
  Product6/1 -> V3/1
  Vamp/1 -> Product5/1, Product2/1, Product6/1

== system hybrid_power/Wind Power System/Wind Turbine/cp(lambda,beta) ==
  lambda : Inport
  beta : Inport  Port=2
  Fcn : Fcn  Expr=1/(1/(u[1]+0.08*u[2])-0.035/(u[2]^3+1))
  Fcn1 : Fcn  Expr=c1*(c2/u[2]-c3*u[3]-c4)*exp(-c5/u[2])+c6*u[1]
  Mux : Mux  Inputs=2
  Mux1 : Mux  Inputs=3
  cp : Outport
  wires:
  Fcn/1 -> Mux1/2  "lambda_i"
  Fcn1/1 -> cp/1
  lambda/1 -> Mux1/1, Mux/1
  Mux1/1 -> Fcn1/1
  beta/1 -> Mux1/3, Mux/2
  Mux/1 -> Fcn/1
